simulink model "driveTrain_PID_controller"  (R2023b)
settings: Solver=VariableStepAuto  StartTime=0.0  StopTime=10  RelTol=1e-3
values from neighbouring files (symbols this model uses):
  b_fr = 0.0016    [modelInit_1FT7042.m]
  D_S = 0.0548    [modelInit_1FT7042.m]
  J_m = 2.81e-4 + 5.5e-4    (= 0.000831)    [modelInit_1FT7042.m]
  k_pos = 1.35    [modelInit_1FT7042.m]
  K_S = 32.94    [modelInit_1FT7042.m]
  k_vel = 1.453488372 * 2.45 * 0.99    (= 3.52543604629)    [modelInit_1FT7042.m]
  N = 1    [modelInit_1FT7042.m]
  omega_step_true = 1    [modelInit_1FT7042.m]
  T_C = (0.0223 + 0.0232) / 2    (= 0.02275)    [modelInit_1FT7042.m]
  T_log = T_s    (= 0.000125)    [modelInit_1FT7042.m]
  T_s = 0.125/1000    (= 0.000125)    [modelInit_1FT7042.m]
  T_S = (0.0441 + 0.0453) / 2    (= 0.0447)    [modelInit_1FT7042.m]
  tau_i = k_vel/k_i    (= 13.6782295038)    [modelInit_1FT7042.m]
  theta_step_true = 0    [modelInit_1FT7042.m]
  theta_true = 1    [modelInit_1FT7042.m]
  x_0 = [0,0]    [modelInit_1FT7042.m]
  x_l_0 = [0,0]    [modelInit_1FT7042.m]
  xf = 1    [modelInit_1FT7042.m]
undefined symbols (not defined in the file or in its folder): J_l
settings Model: Creator=dimpa  LastModifiedBy=amaln
settings SolverCC: MaxConsecutiveMinStep=1000
settings DebuggingCC: UnconnectedInputMsg=warning  UnconnectedOutputMsg=warning  UnconnectedLineMsg=warning
settings ModelReferenceCC: EnableRefExpFcnMdlSchedulingChecks=on
settings RTWCC: DLArmComputeVersion=19.05

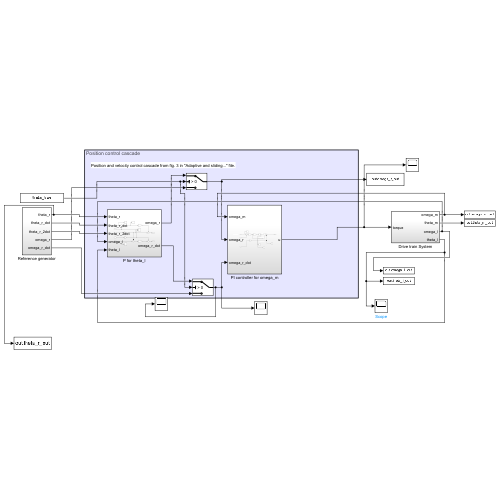
[thumbnail: Simulink's stored preview of the top-level diagram]
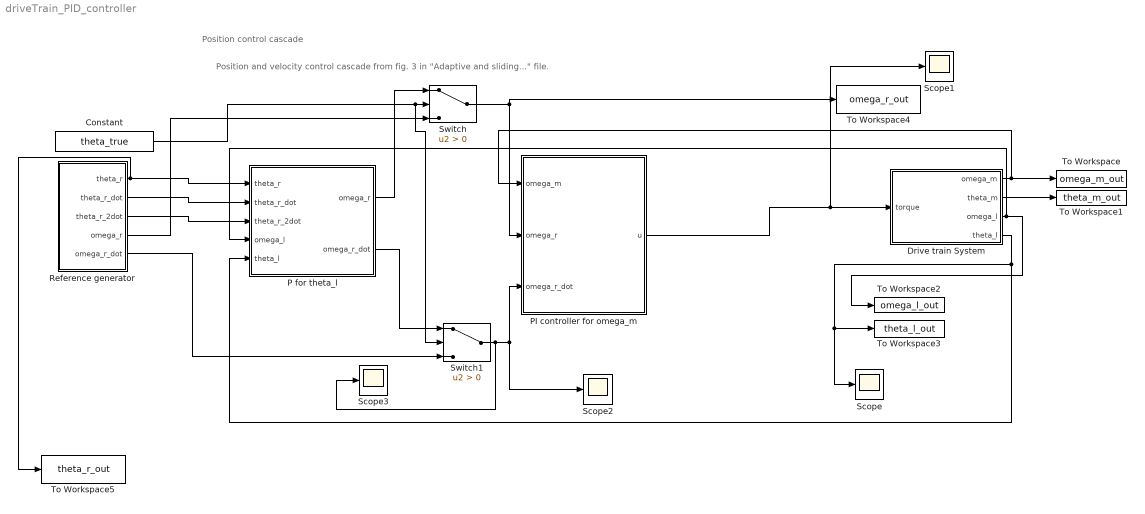
== system driveTrain_PID_controller ==
  note: Position control cascade
  note: Position and velocity control cascade from fig. 3 in "Adaptive and sliding..." file.
  Constant : Constant  Value=theta_true
  Drive train System : Subsystem
  P for theta_l : Subsystem
  PI controller for omega_m : Subsystem
  Reference generator : Subsystem
  Scope{,1..3} (4 alike) : Scope
  Switch : Switch  Criteria=u2 > Threshold  SaturateOnIntegerOverflow=off  InputSameDT=off
  Switch1 : Switch  Criteria=u2 > Threshold  SaturateOnIntegerOverflow=off  InputSameDT=off
  To Workspace : ToWorkspace  VariableName=omega_m_out  SaveFormat=Timeseries  SampleTime=-1
  To Workspace1 : ToWorkspace  VariableName=theta_m_out  SaveFormat=Timeseries  SampleTime=-1
  To Workspace2 : ToWorkspace  VariableName=omega_l_out  SaveFormat=Timeseries  SampleTime=-1
  To Workspace3 : ToWorkspace  VariableName=theta_l_out  SaveFormat=Timeseries  SampleTime=-1
  To Workspace4 : ToWorkspace  VariableName=omega_r_out  SaveFormat=Timeseries  SampleTime=-1
  To Workspace5 : ToWorkspace  VariableName=theta_r_out  SaveFormat=Timeseries  SampleTime=-1
  wires:
  PI controller for omega_m/1(u) -> Scope1/1, Drive train System/1(torque)
  Drive train System/4(theta_l) -> P for theta_l/5(theta_l), Scope/1, To Workspace3/1
  Drive train System/3(omega_l) -> To Workspace2/1, P for theta_l/4(omega_l)
  Drive train System/2(theta_m) -> To Workspace1/1
  Drive train System/1(omega_m) -> PI controller for omega_m/1(omega_m), To Workspace/1
  Constant/1 -> Switch1/2, Switch/2
  Switch/1 -> PI controller for omega_m/2(omega_r), To Workspace4/1
  Switch1/1 -> Scope3/1, Scope2/1, PI controller for omega_m/3(omega_r_dot)
  Reference generator/1(theta_r) -> To Workspace5/1, P for theta_l/1(theta_r)
  Reference generator/2(theta_r_dot) -> P for theta_l/2(theta_r_dot)
  Reference generator/3(theta_r_2dot) -> P for theta_l/3(theta_r_2dot)
  Reference generator/4(omega_r) -> Switch/3
  P for theta_l/1(omega_r) -> Switch/1
  Reference generator/5(omega_r_dot) -> Switch1/3
  P for theta_l/2(omega_r_dot) -> Switch1/1

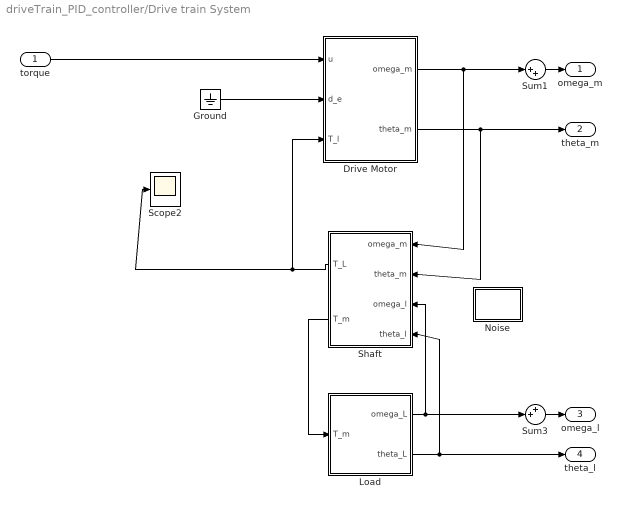
== system driveTrain_PID_controller/Drive train System ==
  torque : Inport
  Drive Motor : Subsystem
  Ground : Ground
  Load : Subsystem
  Noise : Subsystem
  Scope2 : Scope
  Shaft : Subsystem
  Sum1 : Sum  Inputs=|++
  Sum3 : Sum  Inputs=++|
  omega_m : Outport
  theta_m : Outport  Port=2
  omega_l : Outport  Port=3
  theta_l : Outport  Port=4
  wires:
  torque/1 -> Drive Motor/1(u)
  Drive Motor/1(omega_m) -> Sum1/1, Shaft/1(omega_m)
  Shaft/1(T_L) -> Drive Motor/3(T_l), Scope2/1
  Ground/1 -> Drive Motor/2(d_e)
  Load/1(omega_L) -> Sum3/2, Shaft/3(omega_l)
  Shaft/2(T_m) -> Load/1(T_m)
  Sum1/1 -> omega_m/1
  Drive Motor/2(theta_m) -> theta_m/1, Shaft/2(theta_m)
  Sum3/1 -> omega_l/1
  Load/2(theta_L) -> theta_l/1, Shaft/4(theta_l)

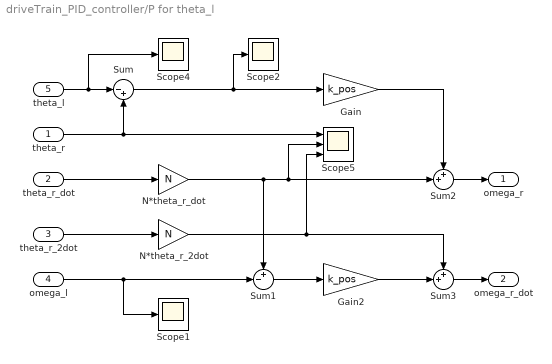
== system driveTrain_PID_controller/P for theta_l ==
  theta_r : Inport
  theta_r_dot : Inport  Port=2
  theta_r_2dot : Inport  Port=3
  omega_l : Inport  Port=4
  theta_l : Inport  Port=5
  Gain : Gain  Gain=k_pos
  Gain2 : Gain  Gain=k_pos
  N*theta_r_2dot : Gain  Gain=N
  N*theta_r_dot : Gain  Gain=N
  Scope1 : Scope
  Scope2 : Scope
  Scope4 : Scope
  Scope5 : Scope  NumInputPorts=3
  Sum : Sum  Inputs=|-+
  Sum1 : Sum  Inputs=+-|
  Sum2 : Sum  Inputs=++|
  Sum3 : Sum  Inputs=++|
  omega_r : Outport
  omega_r_dot : Outport  Port=2
  wires:
  Gain/1 -> Sum2/1
  Sum3/1 -> omega_r_dot/1
  Sum/1 -> Scope2/1, Gain/1
  omega_l/1 -> Sum1/2, Scope1/1
  Sum2/1 -> omega_r/1
  Sum1/1 -> Gain2/1
  Gain2/1 -> Sum3/2
  N*theta_r_dot/1 -> Sum2/2, Scope5/2, Sum1/1
  theta_l/1 -> Scope4/1, Sum/1
  theta_r/1 -> Scope5/1, Sum/2
  theta_r_dot/1 -> N*theta_r_dot/1
  theta_r_2dot/1 -> N*theta_r_2dot/1
  N*theta_r_2dot/1 -> Scope5/3, Sum3/1

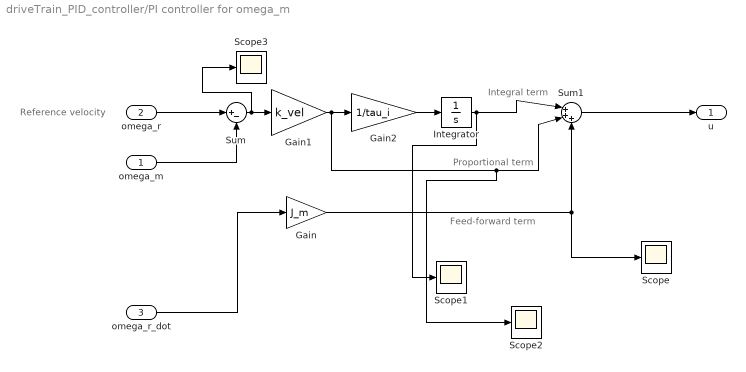
== system driveTrain_PID_controller/PI controller for omega_m ==
  note: Reference velocity
  note: Integral term
  note: Proportional term
  note: Feed-forward term
  omega_m : Inport
  omega_r : Inport  Port=2
  omega_r_dot : Inport  Port=3
  Gain : Gain  Gain=J_m
  Gain1 : Gain  Gain=k_vel
  Gain2 : Gain  Gain=1/tau_i
  Integrator : Integrator
  Scope{,1..3} (4 alike) : Scope
  Sum : Sum  Inputs=|+-
  Sum1 : Sum  Inputs=|+++
  u : Outport
  wires:
  omega_r/1 -> Sum/1
  Sum/1 -> Scope3/1, Gain1/1
  Gain1/1 -> Scope2/1, Sum1/2, Gain2/1
  omega_m/1 -> Sum/2
  Gain2/1 -> Integrator/1
  Integrator/1 -> Scope1/1, Sum1/1
  Sum1/1 -> u/1
  omega_r_dot/1 -> Gain/1
  Gain/1 -> Scope/1, Sum1/3

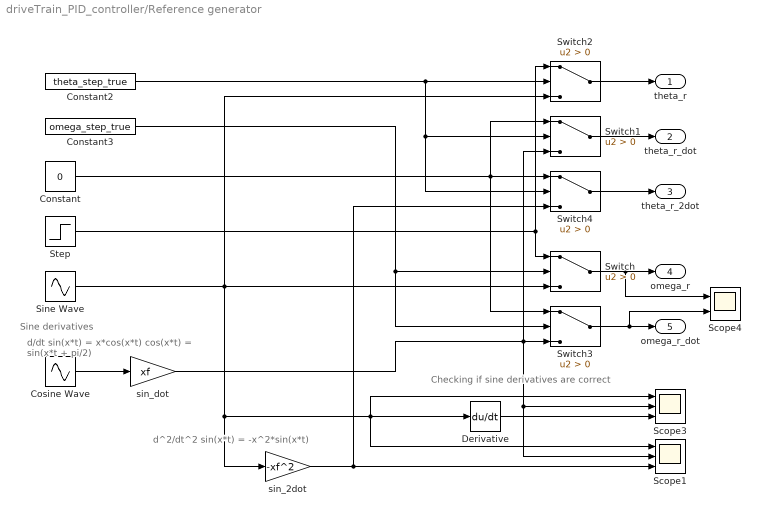
== system driveTrain_PID_controller/Reference generator ==
  note: Sine derivatives
  note: d^2/dt^2 sin(x*t) = -x^2*sin(x*t)
  note: d/dt sin(x*t) = x*cos(x*t)
      |
      |
      |
      |
      | cos(x*t) = sin(x*t + pi/2)
  note: Checking if sine derivatives are correct
  Constant : Constant  Value=0
  Constant2 : Constant  Value=theta_step_true
  Constant3 : Constant  Value=omega_step_true
  Cosine Wave : Sin  Frequency=xf  Phase=pi/2  SampleTime=0
  Derivative : Derivative  CoefficientInTFapproximation=1/100
  Scope1 : Scope  NumInputPorts=3
  Scope3 : Scope  NumInputPorts=3
  Scope4 : Scope  NumInputPorts=2
  Sine Wave : Sin  Frequency=xf  SampleTime=0
  Step : Step  SampleTime=0
  Switch{,1..4} (5 alike) : Switch  Criteria=u2 > Threshold  SaturateOnIntegerOverflow=off  InputSameDT=off
  sin_2dot : Gain  Gain=-xf^2
  sin_dot : Gain  Gain=xf
  theta_r : Outport
  theta_r_dot : Outport  Port=2
  theta_r_2dot : Outport  Port=3
  omega_r : Outport  Port=4
  omega_r_dot : Outport  Port=5
  wires:
  Switch2/1 -> theta_r/1
  Switch/1 -> Scope4/1, omega_r/1
  Switch3/1 -> Scope4/2, omega_r_dot/1
  Cosine Wave/1 -> sin_dot/1
  Switch1/1 -> theta_r_dot/1
  Switch4/1 -> theta_r_2dot/1
  Constant2/1 -> Switch2/2, Switch1/2, Switch4/2
  Constant3/1 -> Switch/2, Switch3/2
  Step/1 -> Switch2/1, Switch/1
  Constant/1 -> Switch3/1, Switch4/1, Switch1/1
  sin_dot/1 -> Scope1/2, Scope3/2, Switch3/3, Switch1/3
  sin_2dot/1 -> Switch4/3, Scope1/3
  Derivative/1 -> Scope3/3
  Sine Wave/1 -> Scope3/1, Scope1/1, Derivative/1, sin_2dot/1, Switch/3, Switch2/3

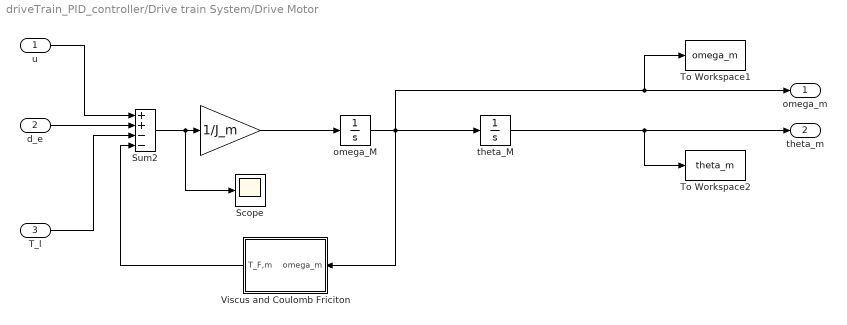
== system driveTrain_PID_controller/Drive train System/Drive Motor ==
  u : Inport
  d_e : Inport  Port=2
  T_l : Inport  Port=3
  "              " : Gain  Gain=1/J_m
  Scope : Scope
  Sum2 : Sum  Inputs=++--
  To Workspace1 : ToWorkspace  VariableName=omega_m  SaveFormat=Timeseries  SampleTime=T_s
  To Workspace2 : ToWorkspace  VariableName=theta_m  SaveFormat=Timeseries  SampleTime=T_s
  Viscus and Coulomb Friciton : Subsystem
  omega_M : Integrator  InitialCondition=x_0(1)
  theta_M : Integrator  InitialCondition=x_0(2)
  omega_m : Outport
  theta_m : Outport  Port=2
  wires:
  "              "/1 -> omega_M/1
  omega_M/1 -> Viscus and Coulomb Friciton/1(omega_m), theta_M/1, To Workspace1/1, omega_m/1
  u/1 -> Sum2/1
  Sum2/1 -> Scope/1, "              "/1
  theta_M/1 -> To Workspace2/1, theta_m/1
  d_e/1 -> Sum2/2
  Viscus and Coulomb Friciton/1(T_F,m) -> Sum2/4
  T_l/1 -> Sum2/3

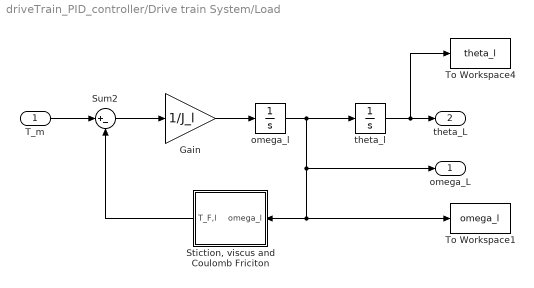
== system driveTrain_PID_controller/Drive train System/Load ==
  T_m : Inport
  Gain : Gain  Gain=1/J_l
  "Stiction, viscus and Coulomb Friciton" : Subsystem
  Sum2 : Sum  Inputs=|+-
  To Workspace1 : ToWorkspace  VariableName=omega_l  SaveFormat=Timeseries  SampleTime=T_log
  To Workspace4 : ToWorkspace  VariableName=theta_l  SaveFormat=Timeseries  SampleTime=T_log
  omega_l : Integrator  InitialCondition=x_l_0(1)
  theta_l : Integrator  InitialCondition=x_l_0(2)
  omega_L : Outport
  theta_L : Outport  Port=2
  wires:
  omega_l/1 -> "Stiction, viscus and Coulomb Friciton"/1(omega_l), To Workspace1/1, omega_L/1, theta_l/1
  theta_l/1 -> To Workspace4/1, theta_L/1
  Sum2/1 -> Gain/1
  Gain/1 -> omega_l/1
  T_m/1 -> Sum2/1
  "Stiction, viscus and Coulomb Friciton"/1(T_F,l) -> Sum2/2

== system driveTrain_PID_controller/Drive train System/Noise ==

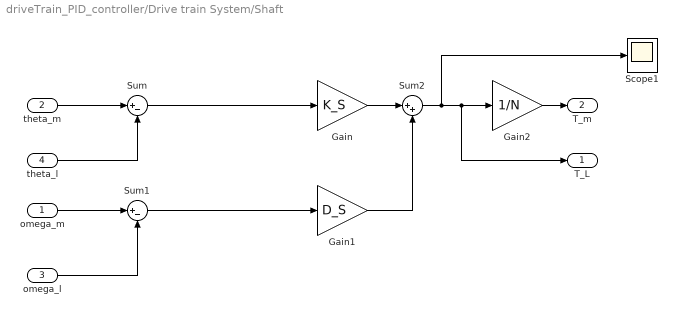
== system driveTrain_PID_controller/Drive train System/Shaft ==
  omega_m : Inport
  theta_m : Inport  Port=2
  omega_l : Inport  Port=3
  theta_l : Inport  Port=4
  Gain : Gain  Gain=K_S
  Gain1 : Gain  Gain=D_S
  Gain2 : Gain  Gain=1/N
  Scope1 : Scope
  Sum : Sum  Inputs=|+-
  Sum1 : Sum  Inputs=|+-
  Sum2 : Sum  Inputs=|++
  T_L : Outport
  T_m : Outport  Port=2
  wires:
  theta_m/1 -> Sum/1
  theta_l/1 -> Sum/2
  omega_m/1 -> Sum1/1
  omega_l/1 -> Sum1/2
  Gain/1 -> Sum2/1
  Gain1/1 -> Sum2/2
  Sum2/1 -> Gain2/1, T_L/1, Scope1/1
  Sum/1 -> Gain/1
  Sum1/1 -> Gain1/1
  Gain2/1 -> T_m/1

== system driveTrain_PID_controller/Drive train System/Drive Motor/Viscus and Coulomb Friciton ==
  omega_m : Inport
  Viscus and Coulomb friction : Subsystem
  T_F,m : Outport
  wires:
  omega_m/1 -> Viscus and Coulomb friction/1(omega)
  Viscus and Coulomb friction/1(T_F,C) -> T_F,m/1

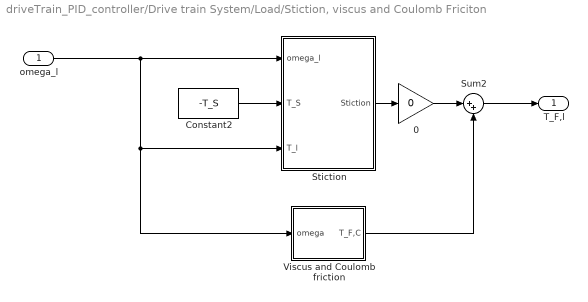
== system driveTrain_PID_controller/Drive train System/Load/Stiction, viscus and Coulomb Friciton ==
  omega_l : Inport
  0 : Gain  Gain=0
  Constant2 : Constant  Value=-T_S
  Stiction : Subsystem
  Sum2 : Sum  Inputs=|++
  Viscus and Coulomb friction : Subsystem
  T_F,l : Outport
  wires:
  Stiction/1(Stiction) -> 0/1
  omega_l/1 -> Stiction/3(T_l), Viscus and Coulomb friction/1(omega), Stiction/1(omega_l)
  Sum2/1 -> T_F,l/1
  Constant2/1 -> Stiction/2(T_S)
  Viscus and Coulomb friction/1(T_F,C) -> Sum2/2
  0/1 -> Sum2/1

== system driveTrain_PID_controller/Drive train System/Drive Motor/Viscus and Coulomb Friciton/Viscus and Coulomb friction ==
  omega : Inport
  Sum2 : Sum  Inputs=|++
  T_c : Gain  Gain=T_C
  b_fr : Gain  Gain=b_fr
  sgn(.) : Subsystem
  T_F,C : Outport
  wires:
  b_fr/1 -> Sum2/1
  T_c/1 -> Sum2/2
  Sum2/1 -> T_F,C/1
  omega/1 -> sgn(.)/1(In1), b_fr/1
  sgn(.)/1(Out1) -> T_c/1

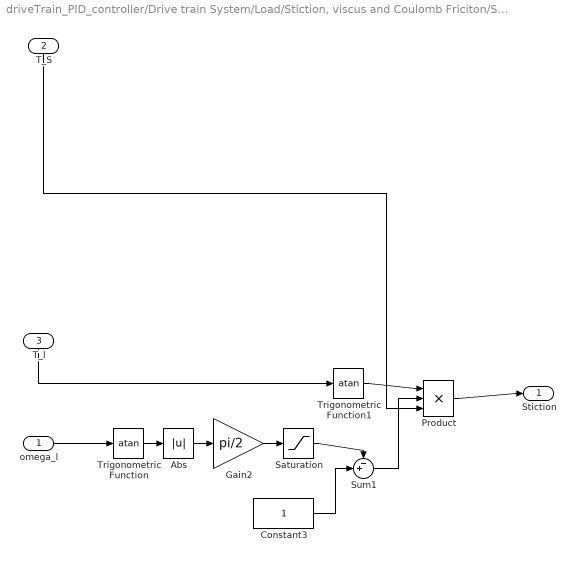
== system driveTrain_PID_controller/Drive train System/Load/Stiction, viscus and Coulomb Friciton/Stiction ==
  omega_l : Inport
  T_S : Inport  Port=2
  T_l : Inport  Port=3
  Abs : Abs  SaturateOnIntegerOverflow=off
  Constant3 : Constant
  Gain2 : Gain  Gain=pi/2
  Product : Product  Inputs=3
  Saturation : Saturate  UpperLimit=1  LowerLimit=0
  Sum1 : Sum  Inputs=-+|
  Trigonometric Function : Trigonometry  Operator=atan
  Trigonometric Function1 : Trigonometry  Operator=atan
  Stiction : Outport
  wires:
  Constant3/1 -> Sum1/2
  Abs/1 -> Gain2/1
  Trigonometric Function/1 -> Abs/1
  Gain2/1 -> Saturation/1
  Sum1/1 -> Product/2
  Product/1 -> Stiction/1
  T_l/1 -> Trigonometric Function1/1
  Trigonometric Function1/1 -> Product/1
  Saturation/1 -> Sum1/1
  T_S/1 -> Product/3
  omega_l/1 -> Trigonometric Function/1

== system driveTrain_PID_controller/Drive train System/Load/Stiction, viscus and Coulomb Friciton/Viscus and Coulomb friction ==
  omega : Inport
  Sum2 : Sum  Inputs=|++
  T_c : Gain  Gain=T_C
  b_fr : Gain  Gain=b_fr
  sgn(.) : Subsystem
  T_F,C : Outport
  wires:
  b_fr/1 -> Sum2/1
  T_c/1 -> Sum2/2
  Sum2/1 -> T_F,C/1
  omega/1 -> sgn(.)/1(In1), b_fr/1
  sgn(.)/1(Out1) -> T_c/1

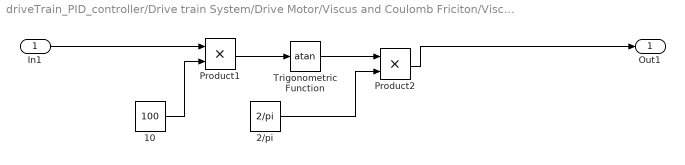
== system driveTrain_PID_controller/Drive train System/Drive Motor/Viscus and Coulomb Friciton/Viscus and Coulomb friction/sgn(.) ==
  In1 : Inport
  10 : Constant  Value=100
  2/pi : Constant  Value=2/pi
  Product1 : Product
  Product2 : Product
  Trigonometric Function : Trigonometry  Operator=atan  SampleTime=T_s
  Out1 : Outport
  wires:
  Trigonometric Function/1 -> Product2/1
  Product2/1 -> Out1/1
  In1/1 -> Product1/1
  10/1 -> Product1/2
  Product1/1 -> Trigonometric Function/1
  2/pi/1 -> Product2/2

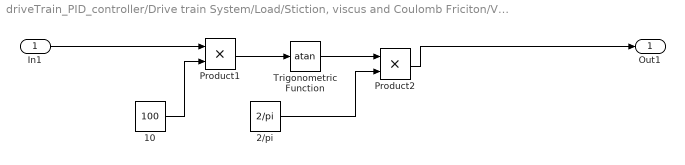
== system driveTrain_PID_controller/Drive train System/Load/Stiction, viscus and Coulomb Friciton/Viscus and Coulomb friction/sgn(.) ==
  In1 : Inport
  10 : Constant  Value=100
  2/pi : Constant  Value=2/pi
  Product1 : Product
  Product2 : Product
  Trigonometric Function : Trigonometry  Operator=atan  SampleTime=T_s
  Out1 : Outport
  wires:
  Trigonometric Function/1 -> Product2/1
  Product2/1 -> Out1/1
  In1/1 -> Product1/1
  10/1 -> Product1/2
  Product1/1 -> Trigonometric Function/1
  2/pi/1 -> Product2/2
